simulink model "loadcell"  (R2024b)
settings: Solver=FixedStepAuto  StartTime=0.0  StopTime=inf  FixedStep=0.1  RelTol=1e-3  EnableMultiTasking=on
libraries: stm32f4xxblockslib x5, dspfdesign x2, dspstat3 x1
settings Model: STM32="{\"AnalogInput\":[{\"ID\":\"loadcell:4\"},{\"ID\":\"loadcell:35\"},{\"ID\":\"loadcell:36\"}],\"DigitalPortRead\":[{\"ID\":\"loadcell:25\"},{\"ID\":\"loadcell:88\"}]}"  Creator=charmil  LastModifiedBy=charmil
settings OptimizationCC: DefaultParameterBehavior=Inlined  EnhancedBackFolding=on  PassReuseOutputArgsAs=Individual arguments  ZeroExternalMemoryAtStartup=off  ZeroInternalMemoryAtStartup=off  MaxStackSize=512  OptimizeBlockOrder=speed  DifferentSizesBufferReuse=on  OptimizationCustomize=off  EfficientTunableParamExpr=on
settings DebuggingCC: ParameterTunabilityLossMsg=error
settings HardwareCC: ProdBitPerPointer=32  ProdBitPerSizeT=32  ProdBitPerPtrDiffT=32  ProdLargestAtomicInteger=Long  ProdLargestAtomicFloat=Double  ProdWordSize=32  ProdLongLongMode=on  ProdHWDeviceType=ARM Compatible->ARM Cortex-M
settings SFSimCC: MATLABDynamicMemAlloc=off
settings RTWCC: Description=Embedded Coder  SystemTargetFile=ert.tlc  HardwareBoard=STM32G4xx Based  TemplateMakefile=ert_default_tmf  Toolchain=GNU Tools for ARM Embedded Processors
settings CodeAppCC: ForceParamTrailComments=on  IgnoreCustomStorageClasses=off  OperatorAnnotations=on  SimulinkDataObjDesc=on  SFDataObjDesc=on  InsertBlockDesc=on
settings ERTTargetCC: TargetLangStandard=C99 (ISO)  CodeReplacementLibrary=ARM Cortex-M  ExtModeTransport=3  ExtModeStaticAlloc=on  ExtModeStaticAllocSize=2048  ExtModeMexFile=ext_xcp  ExtModeIntrfLevel=Level2 - Open

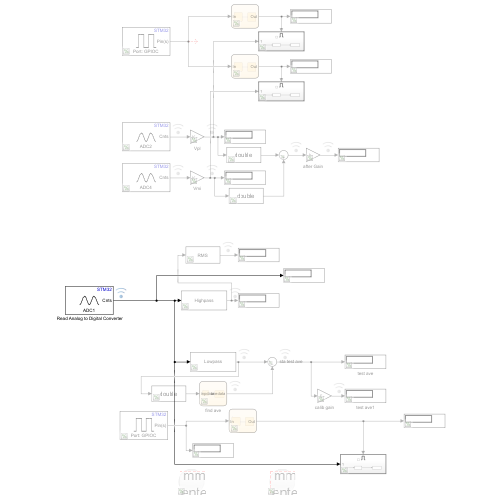
[thumbnail: Simulink's stored preview of the top-level diagram]
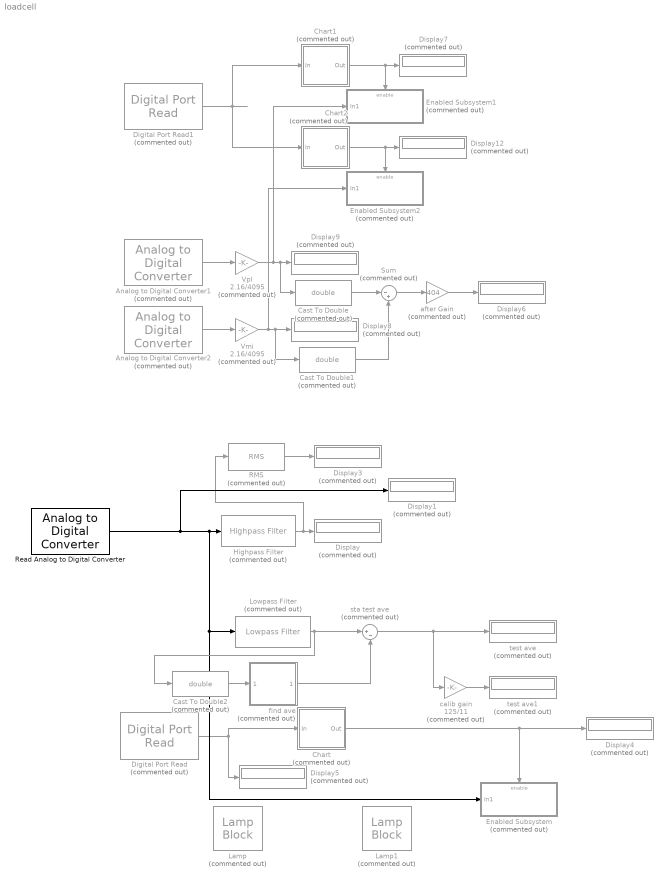
== system loadcell ==
  " Read Analog to Digital Converter" : stm32f4xxblockslib/Analog to Digital Converter  ADCModule=ADC1  ConversionGroup=Regular  TriggerMode=Trigger and read  NumberOfConversions=1  EnableBufferConv=off  BufferLength=1  OutputStatus=off  SampleTime=-1  EnableSimPort=off  hoistedMaskSrc=ECSoC/ECSimCodegen/Analog to Digital Converter
  Analog to Digital Converter1 : stm32f4xxblockslib/Analog to Digital Converter  Commented=on  ADCModule=ADC2  ConversionGroup=Regular  TriggerMode=Trigger and read  NumberOfConversions=1  EnableBufferConv=off  BufferLength=1  OutputStatus=off  SampleTime=-1  EnableSimPort=off  hoistedMaskSrc=ECSoC/ECSimCodegen/Analog to Digital Converter
  Analog to Digital Converter2 : stm32f4xxblockslib/Analog to Digital Converter  Commented=on  ADCModule=ADC4  ConversionGroup=Regular  TriggerMode=Trigger and read  NumberOfConversions=1  EnableBufferConv=off  BufferLength=1  OutputStatus=off  SampleTime=-1  EnableSimPort=off  hoistedMaskSrc=ECSoC/ECSimCodegen/Analog to Digital Converter
  Cast To Double : DataTypeConversion  Commented=on  OutDataTypeStr=double  SaturateOnIntegerOverflow=off  RndMeth=Floor
  Cast To Double1 : DataTypeConversion  Commented=on  OutDataTypeStr=double  SaturateOnIntegerOverflow=off  RndMeth=Floor
  Cast To Double2 : DataTypeConversion  Commented=on  OutDataTypeStr=double  SaturateOnIntegerOverflow=off  RndMeth=Floor
  Chart : Stateflow chart  Commented=on  TreatAsAtomicUnit=on
  Chart1 : Stateflow chart  Commented=on  TreatAsAtomicUnit=on
  Chart2 : Stateflow chart  Commented=on  TreatAsAtomicUnit=on
  Digital Port Read : stm32f4xxblockslib/Digital Port Read  Commented=on  PortName=GPIOC  PinNumber=13  ReadOperation=on  IOAsArray=on  SampleTime=-1  EnableSimPort=off  hoistedMaskSrc=ECSoC/ECSimCodegen/Digital Port Read
      settings: LibrarySourceBlock=stm32g4xxblockslib/Digital Port Read
  Digital Port Read1 : stm32f4xxblockslib/Digital Port Read  Commented=on  PortName=GPIOC  PinNumber=13  ReadOperation=on  IOAsArray=on  SampleTime=-1  EnableSimPort=off  hoistedMaskSrc=ECSoC/ECSimCodegen/Digital Port Read
      settings: LibrarySourceBlock=stm32g4xxblockslib/Digital Port Read
  Display{,1,3..9,12} (10 alike) : Display  Commented=on
  Enabled Subsystem : Subsystem  Commented=on  TreatAsAtomicUnit=on
  Enabled Subsystem1 : Subsystem  Commented=on  TreatAsAtomicUnit=on
  Enabled Subsystem2 : Subsystem  Commented=on  TreatAsAtomicUnit=on
  Highpass Filter : dspfdesign/Highpass Filter  Commented=on  FilterType=FIR  DesignForMinimumOrder=on  FilterOrder=50  StopbandFrequency=0.2  PassbandFrequency=0.3  StopbandAttenuation=80  PassbandRipple=0.1  SampleRateMode=Use normalized frequency (0 to 1)  SampleRate=44100  SimulateUsing=Interpreted execution  roundingMode=Floor  coeffsDataTypeStr=fixdt(1,16)
  Lamp : LampBlock  Commented=on  LabelPosition=Hide
  Lamp1 : LampBlock  Commented=on  LabelPosition=Hide
  Lowpass Filter : dspfdesign/Lowpass Filter  Commented=on  FilterType=FIR  DesignForMinimumOrder=on  FilterOrder=50  PassbandFrequency=0.01  StopbandFrequency=0.15  PassbandRipple=0.1  StopbandAttenuation=80  SampleRateMode=Use normalized frequency (0 to 1)  SampleRate=44100  SimulateUsing=Interpreted execution  roundingMode=Floor  coeffsDataTypeStr=fixdt(1,16)
  RMS : dspstat3/RMS  Commented=on  run=off  directionMode=Each column  dimension=1  InputProcessing=Columns as channels (frame based)  reset_popup=None
  Sum : Sum  Commented=on  Inputs=|-+
  Vmi : Gain  Commented=on  Gain=2.16/4095
  Vpl : Gain  Commented=on  Gain=2.16/4095
  after Gain : Gain  Commented=on  Gain=404
  calib gain : Gain  Commented=on  Gain=125/11
  find ave : Stateflow chart  Commented=on  TreatAsAtomicUnit=on
  sta test ave : Sum  Commented=on  Inputs=|+-
  test ave : Display  Commented=on
  test ave1 : Display  Commented=on
  wires:
  Highpass Filter/1 -> RMS/1, Display/1
  RMS/1 -> Display3/1
  Chart/1(Out) -> Enabled Subsystem/Enable, Display4/1
  Digital Port Read/1 -> Display5/1, Chart/1(In)
  Analog to Digital Converter1/1 -> Vpl/1
  Vpl/1 -> Cast To Double/1, Display9/1, Enabled Subsystem1/1(In1)
  Vmi/1 -> Display8/1, Cast To Double1/1, Enabled Subsystem2/1(In1)
  after Gain/1 -> Display6/1
  Sum/1 -> after Gain/1
  Analog to Digital Converter2/1 -> Vmi/1
  Chart1/1(Out) -> Display7/1, Enabled Subsystem1/Enable
  Chart2/1(Out) -> Display12/1, Enabled Subsystem2/Enable
  Digital Port Read1/1 -> Chart1/1(In), Chart2/1(In)
  Cast To Double/1 -> Sum/1
  Cast To Double1/1 -> Sum/2
  " Read Analog to Digital Converter"/1 -> Display1/1, Enabled Subsystem/1(In1), Lowpass Filter/1, Highpass Filter/1
  sta test ave/1 -> calib gain/1, test ave/1
  Cast To Double2/1 -> find ave/1(inpdata)
  find ave/1(avedata) -> sta test ave/2
  calib gain/1 -> test ave1/1
  Lowpass Filter/1 -> Cast To Double2/1, sta test ave/1

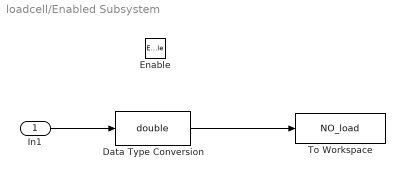
== system loadcell/Enabled Subsystem ==
  In1 : Inport
  Enable : EnablePort
  Data Type Conversion : DataTypeConversion  OutDataTypeStr=double  SaturateOnIntegerOverflow=off  RndMeth=Floor
  To Workspace : ToWorkspace  VariableName=NO_load  SampleTime=-1
      settings: Save2DSignal=2-D array (concatenate along first dimension)
  wires:
  In1/1 -> Data Type Conversion/1
  Data Type Conversion/1 -> To Workspace/1

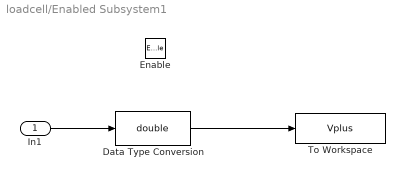
== system loadcell/Enabled Subsystem1 ==
  In1 : Inport
  Enable : EnablePort
  Data Type Conversion : DataTypeConversion  OutDataTypeStr=double  SaturateOnIntegerOverflow=off  RndMeth=Floor
  To Workspace : ToWorkspace  VariableName=Vplus  SampleTime=-1
      settings: Save2DSignal=2-D array (concatenate along first dimension)
  wires:
  In1/1 -> Data Type Conversion/1
  Data Type Conversion/1 -> To Workspace/1

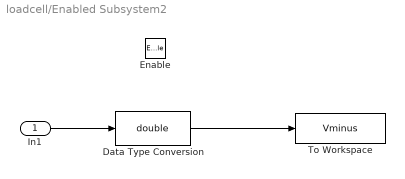
== system loadcell/Enabled Subsystem2 ==
  In1 : Inport
  Enable : EnablePort
  Data Type Conversion : DataTypeConversion  OutDataTypeStr=double  SaturateOnIntegerOverflow=off  RndMeth=Floor
  To Workspace : ToWorkspace  VariableName=Vminus  SampleTime=-1
      settings: Save2DSignal=2-D array (concatenate along first dimension)
  wires:
  In1/1 -> Data Type Conversion/1
  Data Type Conversion/1 -> To Workspace/1

== stateflow chart loadcell/Chart1 ==
  state init
    In;
    Out = 0;
    Count = 1;
  state Log_dtat
    entry:
    during:
    Count = Count + 1;
    Out = 1;
    exit:
    Out = 0;
  (default) -> init
  Log_dtat -> init : [Count > 1000]
  init -> Log_dtat : [In == 1]
  data: In input; Out output; Count local

== stateflow chart loadcell/Chart2 ==
  state init
    In;
    Out = 0;
    Count = 1;
  state Log_dtat
    entry:
    during:
    Count = Count + 1;
    Out = 1;
    exit:
    Out = 0;
  (default) -> init
  Log_dtat -> init : [Count > 1000]
  init -> Log_dtat : [In == 1]
  data: In input; Out output; Count local

== stateflow chart loadcell/Chart ==
  state init
    In;
    Out = 0;
    Count = 1;
  state Log_dtat
    entry:
    during:
    Count = Count + 1;
    Out = 1;
    exit:
    Out = 0;
  (default) -> init
  Log_dtat -> init : [Count > 200]
  init -> Log_dtat : [In == 1]
  data: In input; Out output; Count local

== stateflow chart loadcell/find ave ==
  state sta
    count_data = 0;
    inpdata ;
    avedata ;
    arrdata = 0;
  state summing
    entry:
    during:
    arrdata = arrdata + inpdata;
    count_data = count_data + 1;
    exit:
    avedata = arrdata/50;
  (default) -> sta
  sta -> summing : [(count_data <=0)]
  summing -> sta : [count_data >=50]
  data: inpdata input; count_data local; arrdata local double; avedata output
